simulink model "z53_kaskadaslx"  (R2015a)
settings: Solver=FixedStepDiscrete  StartTime=0.0  StopTime=99.0  FixedStep=1  RelTol=1e-3
settings Model: Creator=Bojana Vasic  LastModifiedBy=Bojana Vasic

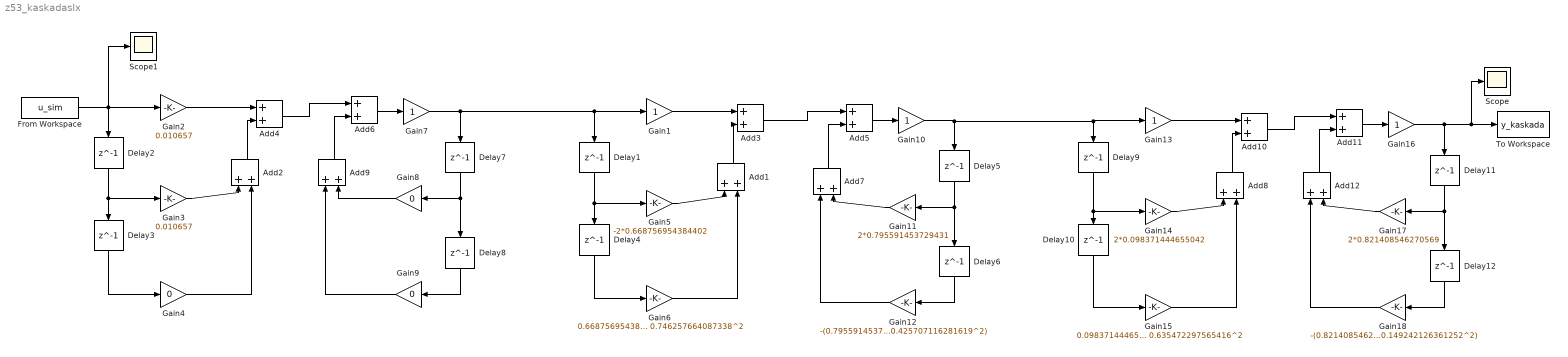
== system z53_kaskadaslx ==
  Add{1..12} (12 alike) : Sum
  Delay{1..12} (12 alike) : Delay  DelayLength=1
  From Workspace : FromWorkspace  VariableName=u_sim  SampleTime=1
  Gain{1,7,10,13,16} (5 alike) : Gain
  Gain11 : Gain  Gain=2*0.795591453729431
  Gain12 : Gain  Gain=-(0.795591453729431^2 + 0.425707116281619^2)
  Gain14 : Gain  Gain=2*0.098371444655042
  Gain15 : Gain  Gain=0.098371444655042^2 + 0.635472297565416^2
  Gain17 : Gain  Gain=2*0.821408546270569
  Gain18 : Gain  Gain=-(0.821408546270569^2 + 0.149242126361252^2)
  Gain2 : Gain  Gain=0.010657
  Gain3 : Gain  Gain=0.010657
  Gain4 : Gain  Gain=0
  Gain5 : Gain  Gain=-2*0.668756954384402
  Gain6 : Gain  Gain=0.668756954384402^2 + 0.746257664087338^2
  Gain8 : Gain  Gain=0
  Gain9 : Gain  Gain=0
  Scope : Scope
  Scope1 : Scope
  To Workspace : ToWorkspace  VariableName=y_kaskada  SampleTime=-1
      settings: Save2DSignal=2-D array (concatenate along first dimension)
  wires:
  From Workspace/1 -> Delay2/1, Scope1/1, Gain2/1
  Delay2/1 -> Gain3/1, Delay3/1
  Gain3/1 -> Add2/1
  Add2/1 -> Add4/2
  Delay3/1 -> Gain4/1
  Gain4/1 -> Add2/2
  Gain8/1 -> Add9/2
  Delay7/1 -> Delay8/1, Gain8/1
  Delay8/1 -> Gain9/1
  Gain9/1 -> Add9/1
  Gain2/1 -> Add4/1
  Add6/1 -> Gain7/1
  Add9/1 -> Add6/2
  Add4/1 -> Add6/1
  Gain7/1 -> Gain1/1, Delay1/1, Delay7/1
  Delay1/1 -> Gain5/1, Delay4/1
  Gain5/1 -> Add1/1
  Add1/1 -> Add3/2
  Delay4/1 -> Gain6/1
  Gain6/1 -> Add1/2
  Gain11/1 -> Add7/2
  Delay5/1 -> Delay6/1, Gain11/1
  Delay6/1 -> Gain12/1
  Gain12/1 -> Add7/1
  Gain1/1 -> Add3/1
  Add5/1 -> Gain10/1
  Add7/1 -> Add5/2
  Add3/1 -> Add5/1
  Gain10/1 -> Gain13/1, Delay9/1, Delay5/1
  Delay9/1 -> Gain14/1, Delay10/1
  Gain14/1 -> Add8/1
  Add8/1 -> Add10/2
  Delay10/1 -> Gain15/1
  Gain15/1 -> Add8/2
  Gain17/1 -> Add12/2
  Delay11/1 -> Delay12/1, Gain17/1
  Delay12/1 -> Gain18/1
  Gain18/1 -> Add12/1
  Gain13/1 -> Add10/1
  Add11/1 -> Gain16/1
  Add12/1 -> Add11/2
  Add10/1 -> Add11/1
  Gain16/1 -> Scope/1, To Workspace/1, Delay11/1
